simulink model "ulise_internal_v0"  (R2025b)
settings: Solver=FixedStepAuto  StartTime=0.0  StopTime=SimSetup.K - 1  FixedStep=1  RelTol=1e-3
InitFcn:
  | InitFcn_ULISE
model workspace (MAT data in the model file):
  Something = 3
undefined symbols (not defined in the file): SimSetup, System, V
libraries: SignalEditorBlockLib x1
settings Model: Creator=savan  LastModifiedBy=daniellawson
settings DebuggingCC: AlgebraicLoopMsg=none

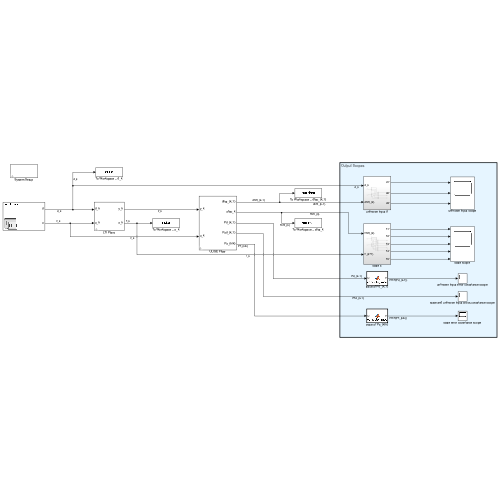
[thumbnail: Simulink's stored preview of the top-level diagram]
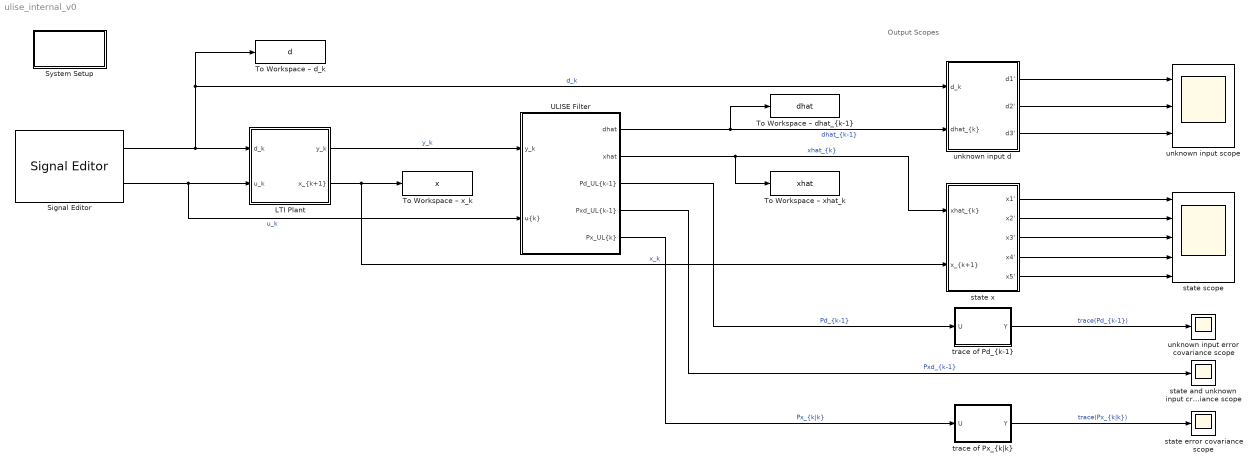
== system ulise_internal_v0 ==
  note: Output Scopes
  LTI Plant : Subsystem  mask{A=System.A, B=System.B, C=System.C, D=System.D, G=System.G, H=System.H, Q=System.Q, R=System.R, InitialState=System.x0, Ts=SimSetup.Ts}
      mask prompts: InitialState "Initial state x_0:"; Ts "Sample Time (-1 for Inherited):"
      mask help:
      | Simulate the states and measurements of a discrete-time, time-invariant linear system of the form:
      |
      | x_{k+1} = A x_k + B u_k + G d_k + w_k,
      | y_k = C x_k + D u_k + H d_k + v_k
      |
      | where x_k is the state vector, u_k is known input vector, d_k is the unknown input vector, y_k is the measurement output vector, w_k is the process noise vector, v_k is the measurement noise vector.
      |
      | Both process noise w_k and measurement noise v_k are zero-mean and uncorrelated, with covariances Q (n-by-n) and R (l-by-l), repsectively.
      mask Help: file:///Users/daniellawson/Documents/Co-op3/Projects/SISE/html/LTI_Plant_Block_overview.html
      mask TypeOptions A: A*x_k multipliation/Gain
      mask TypeOptions B: B*u_k multipliation/Gain
      mask TypeOptions C: C*x_k multipliation/Gain
      mask TypeOptions D: D*u_k multipliation/Gain
      mask TypeOptions G: G*d_k multipliation/Gain
      mask TypeOptions H: H*d_k multipliation/Gain
      mask TypeOptions InitialState: x_{k-1} Delay/InitialCondition
      mask DialogControl DescGroupVar Prompt: Plant
      mask DialogControl ModelParameterContainer Prompt: Model Parameters
      mask DialogControl LTISystemModelContainer Prompt: System Matrices
      mask DialogControl LTISystemNoiseParameters Prompt: Noise Matrices
      mask DialogControl InitialConditions Prompt: Initial Conditions
      mask DialogControl SimulationParameters Prompt: Simulation Paramaters
      mask Display:
      | % Inputs
      | port_label('input', 2, 'u_k');
      | port_label('input', 1, 'd_k');
      | 
      | % Outputs
      | port_label('output', 2, 'x_k');
      | port_label('output', 1, 'y_k');
  Signal Editor : SignalEditorBlockLib/Signal Editor  FileName=ULISE_default_signals.mat  ActiveScenario=input_data  ActiveSignal=d  IsBus=off  OutputBusObjectStr=Bus: BusObject  SampleTime=SimSetup.Ts  Interpolate=off  ZeroCross=off  OutputAfterFinalValue=Holding final value  Unit=inherit  PreserveSignalName=on  ApplySigPropsToAllScenarios=off  ApplySigPropsToAllSignals=off  SignalPropertySource=Signal data in MAT file
  System Setup : Subsystem
      mask help: Describes the files needed to be initialized to use the *LTI Plant* and *ULISE Filter* blocks.
      mask DialogControl ActionsGroupVar Prompt: Actions
      mask DialogControl InitFcnULISEControl Prompt: Open InitFcn_ULISE
      mask DialogControl InitFcnULISEControl Callback: open("./Examples/Simulink/ulise_callbacks/InitFcn_ULISE.m");
  To Workspace – d_k : ToWorkspace  VariableName=d  SaveFormat=Timeseries  SampleTime=-1
  "To Workspace – dhat_{k-1}" : ToWorkspace  VariableName=dhat  SaveFormat=Timeseries  SampleTime=-1
  To Workspace – x_k : ToWorkspace  VariableName=x  SaveFormat=Timeseries  SampleTime=-1
  To Workspace – xhat_k : ToWorkspace  VariableName=xhat  SaveFormat=Timeseries  SampleTime=-1
  ULISE Filter : Subsystem  mask{A=System.A, B=System.B, C=System.C, D=System.D, G=System.G, H=System.H, Q=System.Q, R=System.R, InitialConditionStateEstimate=System.xhat0, InitialConditionStateCov=System.P_x0, Ts=SimSetup.Ts}
      mask prompts: InitialConditionStateEstimate "Initial State Estimate xhat_0:"; InitialConditionStateCov "Initial State Error Covariance Px_0:"; Ts "Sample time (-1 for Inherited):"
      mask help:
      | Estimates the states and unknown inputs of a discrete-time, time-invariant linear system. The states are estimated with a zero-step delay, while the unknown inputs are estimated with a one-step delay.
      |
      | Note: All parameters *must* match the parameters from the LTI Plant Block.
      mask init:
      | %% SVD of H
      | r = rank(H);
      | [U,S,V] = svd(H);
      | U1      = U(:, 1:r); 
      | U2      = U(:, r+1:end);
      | Sigma   = S(1:r, 1:r);
      | V1      = V(:, 1:r);
      | V2      = V(:, r+1:end);
      | 
      | %% Check Assumptions (i) and (ii)
      | 
      | n = size(A,1);
      | p = size(G,2);
      | 
      | if license("test", "Control_Toolbox")
      |     t_zeros = tzero(A,G,C,H)
      |     if rank([A,G;C,H]) ~= n+p
      |         error('Error. System is not strongly detectable.')
      |     end
      |     for i = 1:length(t_zeros)
      |         if abs(t_zeros(i))>1
      |             error('Error. System is not strongly detectable.')
      |         end
      |     end
      | else
      |     warning("Control System Toolbox not available. Condition (i) is not checked.")
      | end
      | 
      | T2 = U2';
      | if rank((T2*C)*(G*V2))<p-r
      |     error('Error. Delay greater or equal to 1. See: Yong, S.Z., Zhu, M., and Frazzoli, E. (2015). Simultaneous input and state estimation with a delay. IEEE Conference on Decision and Control, Osaka, Japan, pp. 468-475')
      | end
      mask TypeOptions InitialConditionStateEstimate: xhat_UL{k} Delay/InitialCondition
      mask TypeOptions InitialConditionStateCov: Px_UL{k} Delay/InitialCondition
      mask DialogControl DescGroupVar Prompt: ULISE Filter
      mask DialogControl ParametersContainer Prompt: Model Parameters
      mask DialogControl ULISESystemModelContainers Prompt: System Matrices
      mask DialogControl ULISENoiseParameters Prompt: Noise Matrices
      mask DialogControl Container6 Prompt: Initial Conditions
      mask DialogControl SimulationParameters Prompt: Simulation Parameters
      mask Display:
      | port_label('input', 2, 'u_k');
      | port_label('input', 1, 'y_k');
      | 
      | port_label('output', 1, 'dhat_{k-1}');
      | port_label('output', 2, 'xhat_k');
      | port_label('output', 3, 'Pd_{k-1}');
      | port_label('output', 4, 'Pxd_{k-1}');
      | port_label('output', 5, 'Px_{k|k}');
  state and unknown input cross-covariance scope : Scope
      settings: ActiveDisplayYMinimum=-5.5275007578366324E+6  ActiveDisplayYMaximum=947500.93266973447
  state error covariance scope : Scope
      settings: ActiveDisplayYMinimum=-621249.98507447576  ActiveDisplayYMaximum=5.5912518070209688E+6  DataLoggingVariableName=ScopeData2
  state scope : Scope  NumInputPorts=5
      settings: ActiveDisplayString=5  ActiveDisplayYMinimum=-0.046170913451183529  ActiveDisplayYMaximum=0.12860695128957148  YLabel=x_5  DataLoggingVariableName=ScopeData7
  state x : Subsystem
  "trace of Pd_{k-1}" : MATLAB Function  TreatAsAtomicUnit=on
  "trace of Px_{k|k}" : MATLAB Function  TreatAsAtomicUnit=on
  unknown input d : Subsystem
  unknown input error covariance scope : Scope
      settings: ActiveDisplayYMinimum=-632500.05670639849  ActiveDisplayYMaximum=5.6925026344334474E+6
  unknown input scope : Scope  NumInputPorts=3
      settings: ActiveDisplayString=3  ActiveDisplayYMinimum=-4.87615367917137  ActiveDisplayYMaximum=4.9009644571376381  YLabel=d_3  DataLoggingVariableName=ScopeData8
  wires:
  ULISE Filter/1(dhat) -> "To Workspace – dhat_{k-1}"/1, unknown input d/2("dhat_{k}")  "dhat_{k-1}"
  Signal Editor/2 -> ULISE Filter/2("u{k}"), LTI Plant/2(u_k)  "u_k"
  Signal Editor/1 -> To Workspace – d_k/1, unknown input d/1(d_k), LTI Plant/1(d_k)  "d_k"
  unknown input d/3(d3') -> unknown input scope/3
  state x/1(x1') -> state scope/1
  state x/3(x3') -> state scope/3
  state x/2(x2') -> state scope/2
  LTI Plant/1(y_k) -> ULISE Filter/1(y_k)  "y_k"
  state x/5(x5') -> state scope/5
  LTI Plant/2("x_{k+1}") -> To Workspace – x_k/1, state x/2("x_{k+1}")  "x_k"
  ULISE Filter/2(xhat) -> To Workspace – xhat_k/1, state x/1("xhat_{k}")  "xhat_{k}"
  unknown input d/1(d1') -> unknown input scope/1
  unknown input d/2(d2') -> unknown input scope/2
  state x/4(x4') -> state scope/4
  ULISE Filter/3("Pd_UL{k-1}") -> "trace of Pd_{k-1}"/1(U)  "Pd_{k-1}"
  ULISE Filter/4("Pxd_UL{k-1}") -> state and unknown input cross-covariance scope/1  "Pxd_{k-1}"
  ULISE Filter/5("Px_UL{k}") -> "trace of Px_{k|k}"/1(U)  "Px_{k|k}"
  "trace of Px_{k|k}"/1(Y) -> state error covariance scope/1  "trace(Px_{k|k})"
  "trace of Pd_{k-1}"/1(Y) -> unknown input error covariance scope/1  "trace(Pd_{k-1})"

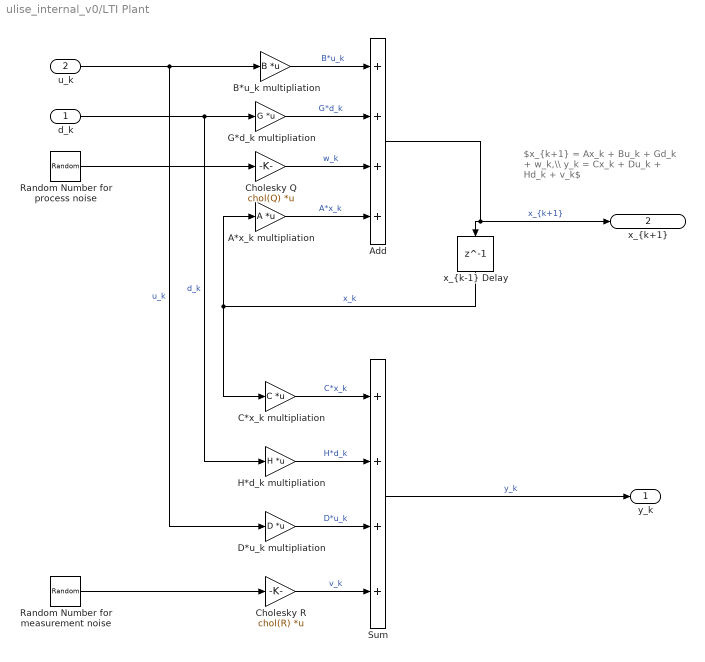
== system ulise_internal_v0/LTI Plant ==
  note: $x_{k+1} = Ax_k + Bu_k + Gd_k + w_k,\\ y_k = Cx_k + Du_k + Hd_k + v_k$
  d_k : Inport
  u_k : Inport  Port=2
  A*x_k multipliation : Gain  Gain=A  Multiplication=Matrix(K*u)
  Add : Sum  Inputs=++++
  B*u_k multipliation : Gain  Gain=B  Multiplication=Matrix(K*u)
  C*x_k multipliation : Gain  Gain=C  Multiplication=Matrix(K*u)
  "Cholesky Q " : Gain  Gain=chol(Q)  Multiplication=Matrix(K*u)
  Cholesky R : Gain  Gain=chol(R)  Multiplication=Matrix(K*u)
  D*u_k multipliation : Gain  Gain=D  Multiplication=Matrix(K*u)
  G*d_k multipliation : Gain  Gain=G  Multiplication=Matrix(K*u)
  H*d_k multipliation : Gain  Gain=H  Multiplication=Matrix(K*u)
  Random Number for measurement noise : RandomNumber  Mean=zeros(size(R,1),1)  Variance=ones(size(R,1),1)  SampleTime=SimSetup.Ts  VectorParams1D=off
  Random Number for process noise : RandomNumber  Mean=zeros(size(Q,1),1)  Variance=ones(size(Q,1),1)  SampleTime=SimSetup.Ts  VectorParams1D=off
  Sum : Sum  Inputs=++++
  "x_{k-1} Delay" : Delay  DelayLength=1  InitialCondition=InitialState
  y_k : Outport
  "x_{k+1}" : Outport  Port=2
  wires:
  D*u_k multipliation/1 -> Sum/3  "D*u_k"
  H*d_k multipliation/1 -> Sum/2  "H*d_k"
  G*d_k multipliation/1 -> Add/2  "G*d_k"
  C*x_k multipliation/1 -> Sum/1  "C*x_k"
  Sum/1 -> y_k/1  "y_k"
  "x_{k-1} Delay"/1 -> A*x_k multipliation/1, C*x_k multipliation/1  "x_k"
  B*u_k multipliation/1 -> Add/1  "B*u_k"
  Add/1 -> "x_{k+1}"/1, "x_{k-1} Delay"/1  "x_{k+1}"
  A*x_k multipliation/1 -> Add/4  "A*x_k"
  d_k/1 -> H*d_k multipliation/1, G*d_k multipliation/1  "d_k"
  u_k/1 -> D*u_k multipliation/1, B*u_k multipliation/1  "u_k"
  Random Number for process noise/1 -> "Cholesky Q "/1
  "Cholesky Q "/1 -> Add/3  "w_k"
  Random Number for measurement noise/1 -> Cholesky R/1
  Cholesky R/1 -> Sum/4  "v_k"

== system ulise_internal_v0/System Setup ==
  note: Edit Initialization Script

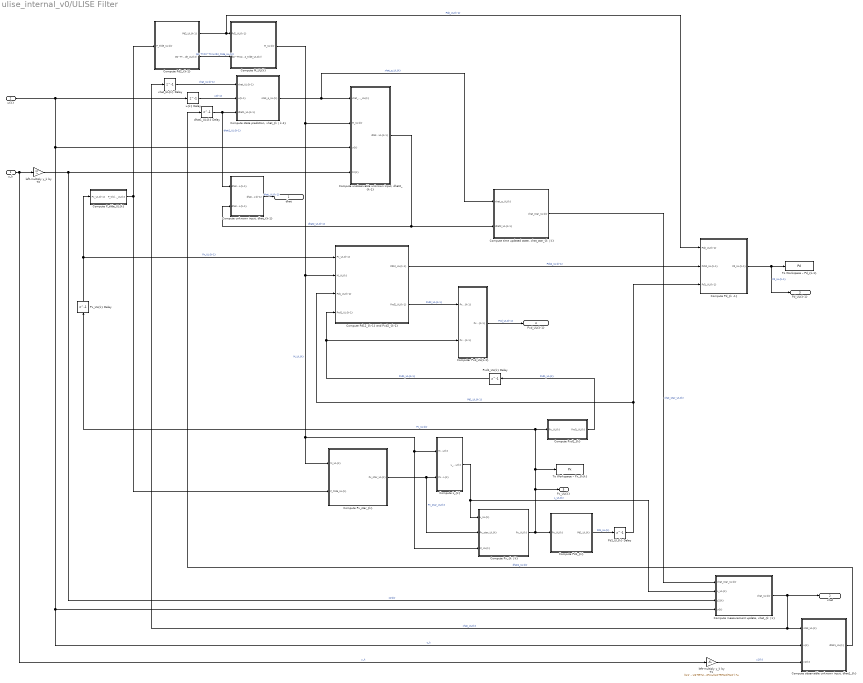
== system ulise_internal_v0/ULISE Filter ==
  y_k : Inport
  "u{k}" : Inport  Port=2
  "Compute L_{k}" : Subsystem
  "Compute M_UL{k}" : Subsystem
  "Compute P_tilde_UL{k}" : Subsystem
  "Compute Pd12_{k-1} and Pxd2_{k-1}" : Subsystem
  "Compute Pd1_{k}" : Subsystem
  "Compute Pd2_{k-1}" : Subsystem
  "Compute Pd_{k -1}" : Subsystem
  "Compute Px_star_{k}" : Subsystem
  "Compute Px_{k | k}" : Subsystem
  "Compute Pxd1_{k}" : Subsystem
  "Compute measurement update, xhat_{k | k}" : Subsystem
  "Compute observable unknown input, dhat1_{k}" : Subsystem
  "Compute state prediction, xhat_{k | k-1} " : Subsystem
  "Compute time updated state, xhat_star_{k | k}" : Subsystem
  "Compute unknown input, dhat_{k-1}" : Subsystem
  "Compute unobservable unknown input, dhat2_{k-1}" : Subsystem
  "Computer Pxd_UL{k-1}" : Subsystem
  "Pd1_UL{k} Delay" : Delay  DelayLength=1
  "Px_UL{k} Delay" : Delay  DelayLength=1  InitialCondition=InitialConditionStateCov  SampleTime=SimSetup.Ts
  "Pxd1_UL{k} Delay" : Delay  DelayLength=1
  "To Workspace – Pd_{k-1}" : ToWorkspace  VariableName=Pd  SaveFormat=Timeseries  SampleTime=-1
  "To Workspace – Px_{k|k}" : ToWorkspace  VariableName=Px  SaveFormat=Timeseries  SampleTime=-1
  "dhat1_UL{k} Delay" : Delay  DelayLength=1  SampleTime=SimSetup.Ts
  left-multiply y_k by T1 : Gain  Gain=(U1' - U1'*R*U2*inv(U2'*R*U2)*U2')  Multiplication=Matrix(K*u)
  "left-multiply y_k by T2 " : Gain  Gain=U2'  Multiplication=Matrix(K*u)
  "u{k} Delay" : Delay  DelayLength=1  SampleTime=SimSetup.Ts
  "xhat_UL{k} Delay" : Delay  DelayLength=1  InitialCondition=InitialConditionStateEstimate  SampleTime=SimSetup.Ts
  dhat : Outport
  xhat : Outport  Port=2
  "Pd_UL{k-1}" : Outport  Port=3
  "Pxd_UL{k-1}" : Outport  Port=4
  "Px_UL{k}" : Outport  Port=5
  wires:
  "Compute Pxd1_{k}"/1("Pxd1_UL{k}") -> "Pxd1_UL{k} Delay"/1  "Pxd1_UL{k}"
  "Compute state prediction, xhat_{k | k-1} "/1("xhat_p_UL{k}") -> "Compute unobservable unknown input, dhat2_{k-1}"/1("xhat_p_UL{k}"), "Compute time updated state, xhat_star_{k | k}"/1("xhat_p_UL{k}")  "xhat_p_UL{k}"
  y_k/1 -> left-multiply y_k by T1/1, "left-multiply y_k by T2 "/1  "y_k"
  left-multiply y_k by T1/1 -> "Compute observable unknown input, dhat1_{k}"/3("z1{k}")  "z1{k}"
  "Compute Pd12_{k-1} and Pxd2_{k-1}"/1("Pd12_UL{k-1}") -> "Compute Pd_{k -1}"/2("Pd12_UL{k-1}")  "Pd12_UL{k-1}"
  "left-multiply y_k by T2 "/1 -> "Compute unobservable unknown input, dhat2_{k-1}"/4("z2{k}"), "Compute measurement update, xhat_{k | k}"/3("z2{k}")  "z2{k}"
  "Compute Pd12_{k-1} and Pxd2_{k-1}"/2("Pxd2_UL{k-1}") -> "Computer Pxd_UL{k-1}"/1("Pxd2_UL{k-1}")  "Pxd2_UL{k-1}"
  "Pd1_UL{k} Delay"/1 -> "Compute Pd_{k -1}"/3("Pd1_UL{k-1}"), "Compute Pd12_{k-1} and Pxd2_{k-1}"/3("Pd1_UL{k-1}")  "Pd1_UL{k-1}"
  "Compute P_tilde_UL{k}"/1("P_tilde_UL{k}") -> "Compute Px_star_{k}"/2("P_tilde_UL{k}"), "Compute Pd2_{k-1}"/1("P_tilde_UL{k}")
  "Pxd1_UL{k} Delay"/1 -> "Compute Pd12_{k-1} and Pxd2_{k-1}"/4("Pxd1_UL{k-1}"), "Computer Pxd_UL{k-1}"/2("Pxd1_UL{k-1}")  "Pxd1_UL{k-1}"
  "Compute M_UL{k}"/1("M_UL{k}") -> "Compute Px_star_{k}"/1("M_UL{k}"), "Compute L_{k}"/1("M_UL{k}"), "Compute Px_{k | k}"/3("M_UL{k}"), "Compute Pd12_{k-1} and Pxd2_{k-1}"/2("M_UL{k}"), "Compute unobservable unknown input, dhat2_{k-1}"/2("M_UL{k}")  "M_UL{k}"
  "Compute Px_star_{k}"/1("Px_star_UL{k}") -> "Compute Px_{k | k}"/2("Px_star_UL{k}"), "Compute L_{k}"/2("Px_star_UL{k}")  "Px_star_UL{k}"
  "Compute Px_{k | k}"/1("Px_UL{k}") -> "Compute Pd1_{k}"/1("Px_UL{k}"), "Px_UL{k}"/1, "Compute Pxd1_{k}"/1("Px_UL{k}"), "Px_UL{k} Delay"/1, "To Workspace – Px_{k|k}"/1  "Px_UL{k}"
  "Compute unknown input, dhat_{k-1}"/1("dhat_UL{k-1}") -> dhat/1  "dhat_UL{k-1}"
  "Compute measurement update, xhat_{k | k}"/1("xhat_UL{k}") -> xhat/1, "xhat_UL{k} Delay"/1, "Compute observable unknown input, dhat1_{k}"/1("xhat_UL{k}")  "xhat_UL{k}"
  "Computer Pxd_UL{k-1}"/1("Pxd_UL{k-1}") -> "Pxd_UL{k-1}"/1  "Pxd_UL{k-1}"
  "Compute Pd2_{k-1}"/1("Pd2_UL{k-1}") -> "Compute Pd_{k -1}"/1("Pd2_UL{k-1}"), "Compute M_UL{k}"/1("Pd2_UL{k-1}")  "Pd2_UL{k-1}"
  "Compute unobservable unknown input, dhat2_{k-1}"/1("dhat2_UL{k-1}") -> "Compute unknown input, dhat_{k-1}"/2("dhat2_UL{k-1}"), "Compute time updated state, xhat_star_{k | k}"/2("dhat2_UL{k-1}")  "dhat2_UL{k-1}"
  "Compute observable unknown input, dhat1_{k}"/1("dhat1_UL{k}") -> "dhat1_UL{k} Delay"/1  "dhat1_UL{k}"
  "dhat1_UL{k} Delay"/1 -> "Compute state prediction, xhat_{k | k-1} "/3("dhat1_UL{k-1}"), "Compute unknown input, dhat_{k-1}"/1("dhat1_UL{k-1}")  "dhat1_UL{k-1}"
  "xhat_UL{k} Delay"/1 -> "Compute state prediction, xhat_{k | k-1} "/1("xhat_UL{k-1}")  "xhat_UL{k-1}"
  "Px_UL{k} Delay"/1 -> "Compute P_tilde_UL{k}"/1("Px_UL{k-1}"), "Compute Pd12_{k-1} and Pxd2_{k-1}"/1("Px_UL{k-1}")  "Px_UL{k-1}"
  "Compute Pd1_{k}"/1("Pd1_UL{k}") -> "Pd1_UL{k} Delay"/1  "Pd1_UL{k}"
  "Compute Pd2_{k-1}"/2("G2^T*C2^T*inv(R2_tilde_UL{k})") -> "Compute M_UL{k}"/2("G2^T*C2^T*inv(R2_tilde_UL{k})")  "G2^T*C2^T*inv(R2_tilde_UL{k})"
  "Compute time updated state, xhat_star_{k | k}"/1("xhat_star_UL{k}") -> "Compute measurement update, xhat_{k | k}"/1("xhat_star_UL{k}")  "xhat_star_UL{k}"
  "u{k}"/1 -> "Compute observable unknown input, dhat1_{k}"/2("u{k}"), "Compute measurement update, xhat_{k | k}"/4("u{k}"), "Compute unobservable unknown input, dhat2_{k-1}"/3("u{k}"), "u{k} Delay"/1  "u_k"
  "Compute L_{k}"/1("L_UL{k}") -> "Compute Px_{k | k}"/1("L_UL{k}"), "Compute measurement update, xhat_{k | k}"/2("L_UL{k}")  "L_UL{k}"
  "Compute Pd_{k -1}"/1("Pd_UL{k-1}") -> "Pd_UL{k-1}"/1, "To Workspace – Pd_{k-1}"/1  "Pd_UL{k-1}"
  "u{k} Delay"/1 -> "Compute state prediction, xhat_{k | k-1} "/2("u{k-1}")  "u{k-1}"

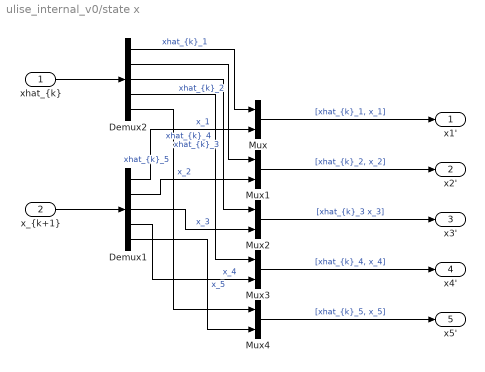
== system ulise_internal_v0/state x ==
  "xhat_{k}" : Inport
  "x_{k+1}" : Inport  Port=2
  Demux1 : Demux  Outputs=5
  Demux2 : Demux  Outputs=5
  Mux{,1..4} (5 alike) : Mux  Inputs=2
  x1' : Outport
  x2' : Outport  Port=2
  x3' : Outport  Port=3
  x4' : Outport  Port=4
  x5' : Outport  Port=5
  wires:
  Mux/1 -> x1'/1  "[xhat_{k}_1, x_1]"
  "xhat_{k}"/1 -> Demux2/1
  Mux4/1 -> x5'/1  "[xhat_{k}_5, x_5]"
  Mux2/1 -> x3'/1  "[xhat_{k}_3 x_3]"
  Demux1/4 -> Mux3/2  "x_4"
  Mux3/1 -> x4'/1  "[xhat_{k}_4, x_4]"
  Mux1/1 -> x2'/1  "[xhat_{k}_2, x_2]"
  Demux1/2 -> Mux1/2  "x_2"
  Demux1/3 -> Mux2/2  "x_3"
  Demux2/5 -> Mux4/1  "xhat_{k}_5"
  Demux2/1 -> Mux/1  "xhat_{k}_1"
  Demux2/4 -> Mux3/1  "xhat_{k}_4"
  Demux2/2 -> Mux1/1  "xhat_{k}_2"
  "x_{k+1}"/1 -> Demux1/1
  Demux1/5 -> Mux4/2  "x_5"
  Demux2/3 -> Mux2/1  "xhat_{k}_3"
  Demux1/1 -> Mux/2  "x_1"

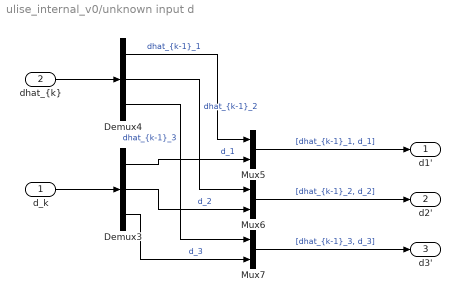
== system ulise_internal_v0/unknown input d ==
  d_k : Inport
  "dhat_{k}" : Inport  Port=2
  Demux3 : Demux  Outputs=3
  Demux4 : Demux  Outputs=3
  Mux5 : Mux  Inputs=2
  Mux6 : Mux  Inputs=2
  Mux7 : Mux  Inputs=2
  d1' : Outport
  d2' : Outport  Port=2
  d3' : Outport  Port=3
  wires:
  Mux6/1 -> d2'/1  "[dhat_{k-1}_2, d_2]"
  d_k/1 -> Demux3/1
  Mux7/1 -> d3'/1  "[dhat_{k-1}_3, d_3]"
  Demux3/3 -> Mux7/2  "d_3"
  Demux4/1 -> Mux5/1  "dhat_{k-1}_1"
  Demux4/2 -> Mux6/1  "dhat_{k-1}_2"
  "dhat_{k}"/1 -> Demux4/1
  Mux5/1 -> d1'/1  "[dhat_{k-1}_1, d_1]"
  Demux3/2 -> Mux6/2  "d_2"
  Demux3/1 -> Mux5/2  "d_1"
  Demux4/3 -> Mux7/1  "dhat_{k-1}_3"

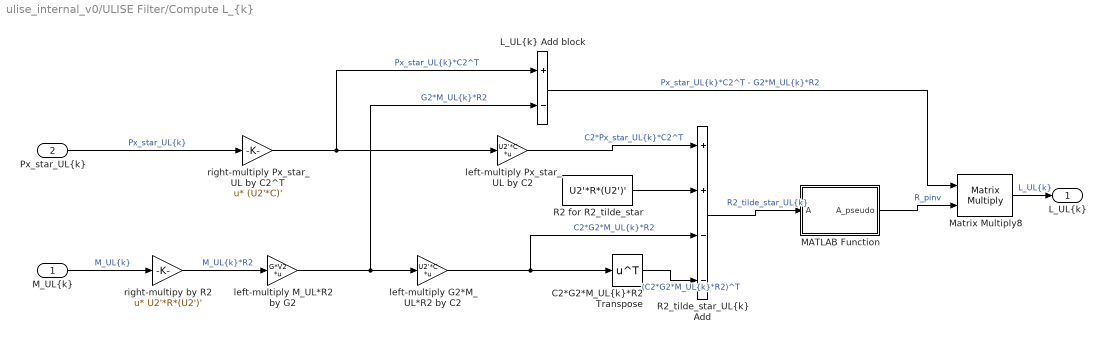
== system ulise_internal_v0/ULISE Filter/Compute L_{k} ==
  "M_UL{k}" : Inport
  "Px_star_UL{k}" : Inport  Port=2
  " R2 for R2_tilde_star" : Constant  Value=U2'*R*(U2')'  VectorParams1D=off  SampleTime=SimSetup.Ts
  "C2*G2*M_UL{k}*R2 Transpose" : Math  Operator=transpose
  "L_UL{k} Add block" : Sum  Inputs=+-
  MATLAB Function : MATLAB Function  TreatAsAtomicUnit=on
  Matrix Multiply8 : Product  Multiplication=Matrix(*)
  "R2_tilde_star_UL{k} Add" : Sum  Inputs=++--
  left-multiply Px_star_UL by C2 : Gain  Gain=U2'*C  Multiplication=Matrix(K*u)
  left-multiply G2*M_UL*R2 by C2 : Gain  Gain=U2'*C  Multiplication=Matrix(K*u)
  left-multiply M_UL*R2 by G2 : Gain  Gain=G*V2  Multiplication=Matrix(K*u)
  "right-multiply Px_star_UL by C2^T " : Gain  Gain=(U2'*C)'  Multiplication=Matrix(u*K)
  right-multipy by R2 : Gain  Gain=U2'*R*(U2')'  Multiplication=Matrix(u*K)
  "L_UL{k}" : Outport
  wires:
  right-multipy by R2/1 -> left-multiply M_UL*R2 by G2/1  "M_UL{k}*R2"
  "Px_star_UL{k}"/1 -> "right-multiply Px_star_UL by C2^T "/1  "Px_star_UL{k}"
  Matrix Multiply8/1 -> "L_UL{k}"/1  "L_UL{k}"
  "right-multiply Px_star_UL by C2^T "/1 -> "L_UL{k} Add block"/1, left-multiply Px_star_UL by C2/1  "Px_star_UL{k}*C2^T"
  left-multiply M_UL*R2 by G2/1 -> left-multiply G2*M_UL*R2 by C2/1, "L_UL{k} Add block"/2  "G2*M_UL{k}*R2"
  "R2_tilde_star_UL{k} Add"/1 -> MATLAB Function/1(A)  "R2_tilde_star_UL{k}"
  left-multiply G2*M_UL*R2 by C2/1 -> "R2_tilde_star_UL{k} Add"/3, "C2*G2*M_UL{k}*R2 Transpose"/1  "C2*G2*M_UL{k}*R2"
  "L_UL{k} Add block"/1 -> Matrix Multiply8/1  "Px_star_UL{k}*C2^T - G2*M_UL{k}*R2"
  " R2 for R2_tilde_star"/1 -> "R2_tilde_star_UL{k} Add"/2
  "M_UL{k}"/1 -> right-multipy by R2/1  "M_UL{k}"
  left-multiply Px_star_UL by C2/1 -> "R2_tilde_star_UL{k} Add"/1  "C2*Px_star_UL{k}*C2^T"
  "C2*G2*M_UL{k}*R2 Transpose"/1 -> "R2_tilde_star_UL{k} Add"/4  "(C2*G2*M_UL{k}*R2)^T"
  MATLAB Function/1(A_pseudo) -> Matrix Multiply8/2  "R_pinv"

== system ulise_internal_v0/ULISE Filter/Compute M_UL{k} ==
  "Pd2_UL{k-1}" : Inport
  "G2^T*C2^T*inv(R2_tilde_UL{k})" : Inport  Port=2
  Matrix Multiply : Product  Multiplication=Matrix(*)
  "M_UL{k}" : Outport
  wires:
  "G2^T*C2^T*inv(R2_tilde_UL{k})"/1 -> Matrix Multiply/2  "G2^T*C2^T*inv(R2_tilde_UL{k})"
  Matrix Multiply/1 -> "M_UL{k}"/1  "M_UL{k}"
  "Pd2_UL{k-1}"/1 -> Matrix Multiply/1  "Pd2_UL{k-1}"

== system ulise_internal_v0/ULISE Filter/Compute P_tilde_UL{k} ==
  "Px_UL{k-1}" : Inport
  Add Qhat : Sum
  Qhat : Constant  Value=G*V1*pinv(Sigma)*((U1' - U1'*R*U2*inv(U2'*R*U2)*U2')*R*(U1' - U1'*R*U2*inv(U2'*R*U2)*U2')')*pinv(Sigma)'*(G*V1)' + Q  VectorParams1D=off  SampleTime=SimSetup.Ts
  left-multiply by Ahat : Gain  Gain=A - G*V1*pinv(Sigma)*((U1' - U1'*R*U2*inv(U2'*R*U2)*U2')*C)  Multiplication=Matrix(K*u)
  right-multiply by Ahat^T : Gain  Gain=(A - G*V1*pinv(Sigma)*((U1' - U1'*R*U2*inv(U2'*R*U2)*U2')*C))'  Multiplication=Matrix(u*K)
  "P_tilde_UL{k}" : Outport
  wires:
  Add Qhat/1 -> "P_tilde_UL{k}"/1  "P_tilde_UL{k}"
  "Px_UL{k-1}"/1 -> right-multiply by Ahat^T/1  "Px_UL{k-1}"
  right-multiply by Ahat^T/1 -> left-multiply by Ahat/1  "Px_UL{k-1}*Ahat^T"
  left-multiply by Ahat/1 -> Add Qhat/1  "Ahat*Px_UL{k-1}*Ahat^T"
  Qhat/1 -> Add Qhat/2  "Qhat"

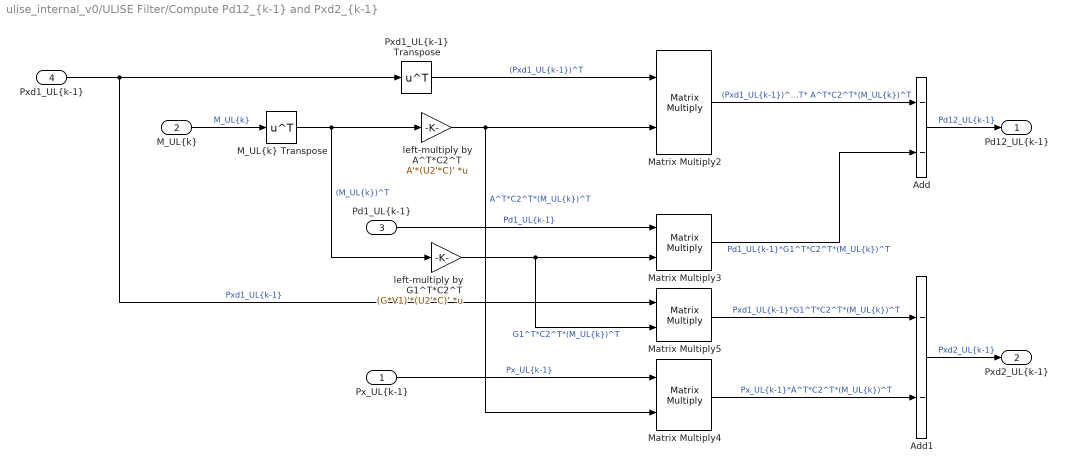
== system ulise_internal_v0/ULISE Filter/Compute Pd12_{k-1} and Pxd2_{k-1} ==
  "Px_UL{k-1}" : Inport
  "M_UL{k}" : Inport  Port=2
  "Pd1_UL{k-1}" : Inport  Port=3
  "Pxd1_UL{k-1}" : Inport  Port=4
  Add : Sum  Inputs=--
  Add1 : Sum  Inputs=--
  "M_UL{k} Transpose" : Math  Operator=transpose
  Matrix Multiply{2..5} (4 alike) : Product  Multiplication=Matrix(*)
  "Pxd1_UL{k-1} Transpose" : Math  Operator=transpose
  left-multiply by A^T*C2^T : Gain  Gain=A'*(U2'*C)'  Multiplication=Matrix(K*u)
  left-multiply by G1^T*C2^T : Gain  Gain=(G*V1)'*(U2'*C)'  Multiplication=Matrix(K*u)
  "Pd12_UL{k-1}" : Outport
  "Pxd2_UL{k-1}" : Outport  Port=2
  wires:
  Add1/1 -> "Pxd2_UL{k-1}"/1  "Pxd2_UL{k-1}"
  left-multiply by A^T*C2^T/1 -> Matrix Multiply2/2, Matrix Multiply4/2  "A^T*C2^T*(M_UL{k})^T"
  Matrix Multiply5/1 -> Add1/1  "Pxd1_UL{k-1}*G1^T*C2^T*(M_UL{k})^T"
  left-multiply by G1^T*C2^T/1 -> Matrix Multiply3/2, Matrix Multiply5/2  "G1^T*C2^T*(M_UL{k})^T"
  Matrix Multiply3/1 -> Add/2  "Pd1_UL{k-1}*G1^T*C2^T*(M_UL{k})^T"
  "M_UL{k}"/1 -> "M_UL{k} Transpose"/1  "M_UL{k}"
  "Pd1_UL{k-1}"/1 -> Matrix Multiply3/1  "Pd1_UL{k-1}"
  Add/1 -> "Pd12_UL{k-1}"/1  "Pd12_UL{k-1}"
  Matrix Multiply4/1 -> Add1/2  "Px_UL{k-1}*A^T*C2^T*(M_UL{k})^T"
  "Px_UL{k-1}"/1 -> Matrix Multiply4/1  "Px_UL{k-1}"
  Matrix Multiply2/1 -> Add/1  "(Pxd1_UL{k-1})^T* A^T*C2^T*(M_UL{k})^T"
  "Pxd1_UL{k-1} Transpose"/1 -> Matrix Multiply2/1  "(Pxd1_UL{k-1})^T"
  "Pxd1_UL{k-1}"/1 -> "Pxd1_UL{k-1} Transpose"/1, Matrix Multiply5/1  "Pxd1_UL{k-1}"
  "M_UL{k} Transpose"/1 -> left-multiply by G1^T*C2^T/1, left-multiply by A^T*C2^T/1  "(M_UL{k})^T"

== system ulise_internal_v0/ULISE Filter/Compute Pd1_{k} ==
  "Px_UL{k}" : Inport
  "R1 " : Constant  Value=(U1' - U1'*R*U2*inv(U2'*R*U2)*U2')*R*(U1' - U1'*R*U2*inv(U2'*R*U2)*U2')'  VectorParams1D=off  SampleTime=SimSetup.Ts
  "R1_tilde_UL{k} Add" : Sum
  "left-multiply Px_UL{k}*C1^T by C1" : Gain  Gain=(U1' - U1'*R*U2*inv(U2'*R*U2)*U2')*C  Multiplication=Matrix(K*u)
  "left-multiply R1_tilde_UL{k}*M1 by M1" : Gain  Gain=pinv(Sigma)  Multiplication=Matrix(K*u)
  "right-multiply Px_UL{k} by C1^T" : Gain  Gain=((U1' - U1'*R*U2*inv(U2'*R*U2)*U2')*C)'  Multiplication=Matrix(u*K)
  "right-multiply R1_tilde_UL{k} by M1" : Gain  Gain=pinv(Sigma)  Multiplication=Matrix(u*K)
  "Pd1_UL{k}" : Outport
  wires:
  "Px_UL{k}"/1 -> "right-multiply Px_UL{k} by C1^T"/1
  "right-multiply Px_UL{k} by C1^T"/1 -> "left-multiply Px_UL{k}*C1^T by C1"/1  "Px_UL{k}*C1^T"
  "right-multiply R1_tilde_UL{k} by M1"/1 -> "left-multiply R1_tilde_UL{k}*M1 by M1"/1  "R1_tilde_UL{k}*M1"
  "left-multiply R1_tilde_UL{k}*M1 by M1"/1 -> "Pd1_UL{k}"/1  "Pd1_UL{k}"
  "left-multiply Px_UL{k}*C1^T by C1"/1 -> "R1_tilde_UL{k} Add"/1  "C1*Px_UL{k}*C1^T"
  "R1_tilde_UL{k} Add"/1 -> "right-multiply R1_tilde_UL{k} by M1"/1  "R1_tilde_UL{k}"
  "R1 "/1 -> "R1_tilde_UL{k} Add"/2

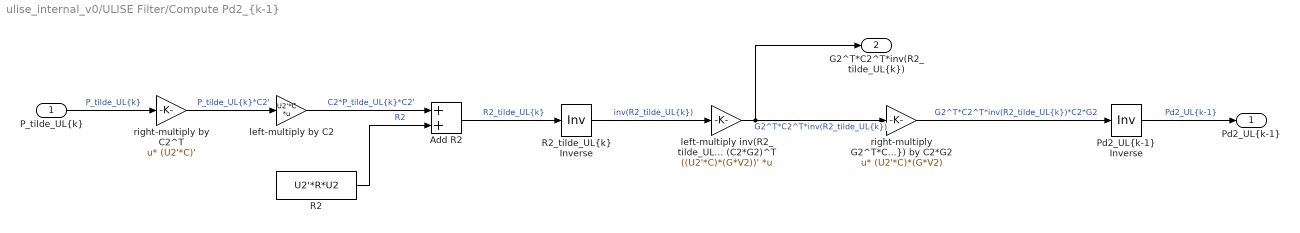
== system ulise_internal_v0/ULISE Filter/Compute Pd2_{k-1} ==
  "P_tilde_UL{k}" : Inport
  Add R2 : Sum
  "Pd2_UL{k-1} Inverse" : Product  Inputs=/  Multiplication=Matrix(*)
  R2 : Constant  Value=U2'*R*U2  VectorParams1D=off  SampleTime=SimSetup.Ts
  "R2_tilde_UL{k} Inverse" : Product  Inputs=/  Multiplication=Matrix(*)
  "left-multiply inv(R2_tilde_UL{k}) by (C2*G2)^T " : Gain  Gain=((U2'*C)*(G*V2))'  Multiplication=Matrix(K*u)
  left-multiply by C2 : Gain  Gain=U2'*C  Multiplication=Matrix(K*u)
  "right-multiply G2^T*C2^T*inv(R2_tilde_UL{k}) by C2*G2" : Gain  Gain=(U2'*C)*(G*V2)  Multiplication=Matrix(u*K)
  right-multiply by C2^T : Gain  Gain=(U2'*C)'  Multiplication=Matrix(u*K)
  "Pd2_UL{k-1}" : Outport
  "G2^T*C2^T*inv(R2_tilde_UL{k})" : Outport  Port=2
  wires:
  left-multiply by C2/1 -> Add R2/1  "C2*P_tilde_UL{k}*C2'"
  "P_tilde_UL{k}"/1 -> right-multiply by C2^T/1  "P_tilde_UL{k}"
  right-multiply by C2^T/1 -> left-multiply by C2/1  "P_tilde_UL{k}*C2'"
  "right-multiply G2^T*C2^T*inv(R2_tilde_UL{k}) by C2*G2"/1 -> "Pd2_UL{k-1} Inverse"/1  "G2^T*C2^T*inv(R2_tilde_UL{k})*C2*G2"
  "R2_tilde_UL{k} Inverse"/1 -> "left-multiply inv(R2_tilde_UL{k}) by (C2*G2)^T "/1  "inv(R2_tilde_UL{k})"
  R2/1 -> Add R2/2  "R2"
  "Pd2_UL{k-1} Inverse"/1 -> "Pd2_UL{k-1}"/1  "Pd2_UL{k-1}"
  Add R2/1 -> "R2_tilde_UL{k} Inverse"/1  "R2_tilde_UL{k}"
  "left-multiply inv(R2_tilde_UL{k}) by (C2*G2)^T "/1 -> "right-multiply G2^T*C2^T*inv(R2_tilde_UL{k}) by C2*G2"/1, "G2^T*C2^T*inv(R2_tilde_UL{k})"/1  "G2^T*C2^T*inv(R2_tilde_UL{k})"

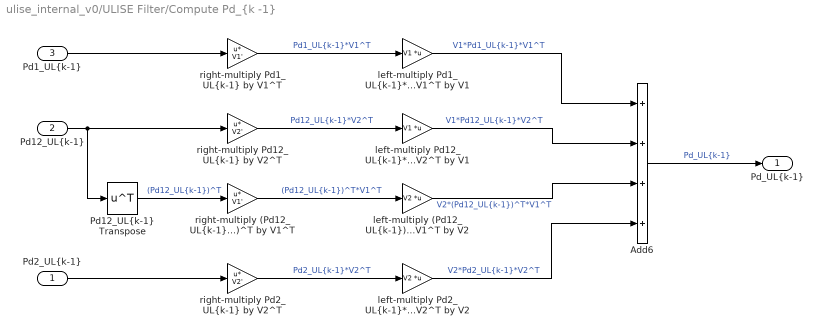
== system ulise_internal_v0/ULISE Filter/Compute Pd_{k -1} ==
  "Pd2_UL{k-1}" : Inport
  "Pd12_UL{k-1}" : Inport  Port=2
  "Pd1_UL{k-1}" : Inport  Port=3
  Add6 : Sum  Inputs=++++
  "Pd12_UL{k-1} Transpose" : Math  Operator=transpose
  "left-multiply (Pd12_UL{k-1})^T*V1^T by V2" : Gain  Gain=V2  Multiplication=Matrix(K*u)
  "left-multiply Pd12_UL{k-1}*V2^T by V1" : Gain  Gain=V1  Multiplication=Matrix(K*u)
  "left-multiply Pd1_UL{k-1}*V1^T by V1" : Gain  Gain=V1  Multiplication=Matrix(K*u)
  "left-multiply Pd2_UL{k-1}*V2^T by V2" : Gain  Gain=V2  Multiplication=Matrix(K*u)
  "right-multiply (Pd12_UL{k-1})^T by V1^T" : Gain  Gain=V1'  Multiplication=Matrix(u*K)
  "right-multiply Pd12_UL{k-1} by V2^T" : Gain  Gain=V2'  Multiplication=Matrix(u*K)
  "right-multiply Pd1_UL{k-1} by V1^T" : Gain  Gain=V1'  Multiplication=Matrix(u*K)
  "right-multiply Pd2_UL{k-1} by V2^T" : Gain  Gain=V2'  Multiplication=Matrix(u*K)
  "Pd_UL{k-1}" : Outport
  wires:
  "Pd2_UL{k-1}"/1 -> "right-multiply Pd2_UL{k-1} by V2^T"/1
  "Pd12_UL{k-1}"/1 -> "right-multiply Pd12_UL{k-1} by V2^T"/1, "Pd12_UL{k-1} Transpose"/1
  "left-multiply Pd12_UL{k-1}*V2^T by V1"/1 -> Add6/2  "V1*Pd12_UL{k-1}*V2^T"
  "Pd1_UL{k-1}"/1 -> "right-multiply Pd1_UL{k-1} by V1^T"/1
  "left-multiply Pd2_UL{k-1}*V2^T by V2"/1 -> Add6/4  "V2*Pd2_UL{k-1}*V2^T"
  "right-multiply Pd12_UL{k-1} by V2^T"/1 -> "left-multiply Pd12_UL{k-1}*V2^T by V1"/1  "Pd12_UL{k-1}*V2^T"
  "left-multiply Pd1_UL{k-1}*V1^T by V1"/1 -> Add6/1  "V1*Pd1_UL{k-1}*V1^T"
  "right-multiply (Pd12_UL{k-1})^T by V1^T"/1 -> "left-multiply (Pd12_UL{k-1})^T*V1^T by V2"/1  "(Pd12_UL{k-1})^T*V1^T"
  Add6/1 -> "Pd_UL{k-1}"/1  "Pd_UL{k-1}"
  "right-multiply Pd1_UL{k-1} by V1^T"/1 -> "left-multiply Pd1_UL{k-1}*V1^T by V1"/1  "Pd1_UL{k-1}*V1^T"
  "right-multiply Pd2_UL{k-1} by V2^T"/1 -> "left-multiply Pd2_UL{k-1}*V2^T by V2"/1  "Pd2_UL{k-1}*V2^T"
  "left-multiply (Pd12_UL{k-1})^T*V1^T by V2"/1 -> Add6/3  "V2*(Pd12_UL{k-1})^T*V1^T"
  "Pd12_UL{k-1} Transpose"/1 -> "right-multiply (Pd12_UL{k-1})^T by V1^T"/1  "(Pd12_UL{k-1})^T"

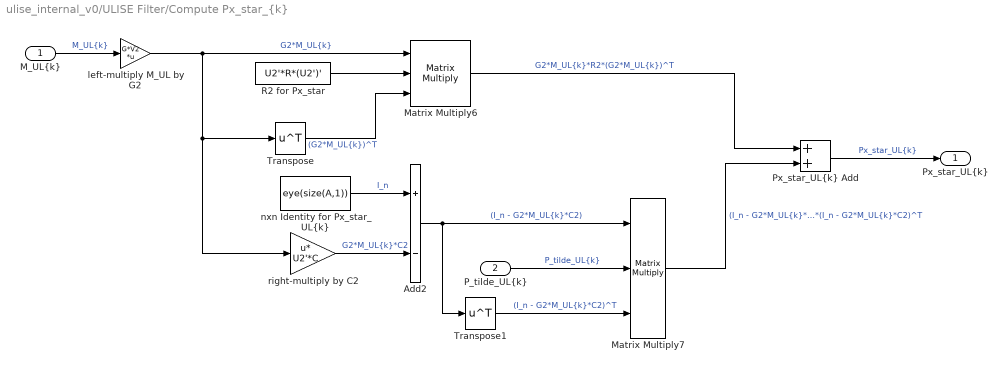
== system ulise_internal_v0/ULISE Filter/Compute Px_star_{k} ==
  "M_UL{k}" : Inport
  "P_tilde_UL{k}" : Inport  Port=2
  " R2 for Px_star" : Constant  Value=U2'*R*(U2')'  SampleTime=SimSetup.Ts
  Add2 : Sum  Inputs=+-
  Matrix Multiply6 : Product  Inputs=3  Multiplication=Matrix(*)
  Matrix Multiply7 : Product  Inputs=3  Multiplication=Matrix(*)
  "Px_star_UL{k} Add" : Sum
  Transpose : Math  Operator=transpose
  Transpose1 : Math  Operator=transpose
  left-multiply M_UL by G2 : Gain  Gain=G*V2  Multiplication=Matrix(K*u)
  "nxn Identity for Px_star_UL{k}" : Constant  Value=eye(size(A,1))  VectorParams1D=off  SampleTime=SimSetup.Ts
  right-multiply by C2 : Gain  Gain=U2'*C  Multiplication=Matrix(u*K)
  "Px_star_UL{k}" : Outport
  wires:
  right-multiply by C2/1 -> Add2/2  "G2*M_UL{k}*C2"
  left-multiply M_UL by G2/1 -> right-multiply by C2/1, Transpose/1, Matrix Multiply6/1  "G2*M_UL{k}"
  Transpose1/1 -> Matrix Multiply7/3  "(I_n - G2*M_UL{k}*C2)^T"
  Matrix Multiply7/1 -> "Px_star_UL{k} Add"/2  "(I_n - G2*M_UL{k}*C2)*P_tilde*(I_n - G2*M_UL{k}*C2)^T"
  " R2 for Px_star"/1 -> Matrix Multiply6/2
  "M_UL{k}"/1 -> left-multiply M_UL by G2/1  "M_UL{k}"
  "P_tilde_UL{k}"/1 -> Matrix Multiply7/2  "P_tilde_UL{k}"
  "Px_star_UL{k} Add"/1 -> "Px_star_UL{k}"/1  "Px_star_UL{k}"
  Add2/1 -> Transpose1/1, Matrix Multiply7/1  "(I_n - G2*M_UL{k}*C2)"
  "nxn Identity for Px_star_UL{k}"/1 -> Add2/1  "I_n"
  Transpose/1 -> Matrix Multiply6/3  "(G2*M_UL{k})^T"
  Matrix Multiply6/1 -> "Px_star_UL{k} Add"/1  "G2*M_UL{k}*R2*(G2*M_UL{k})^T"

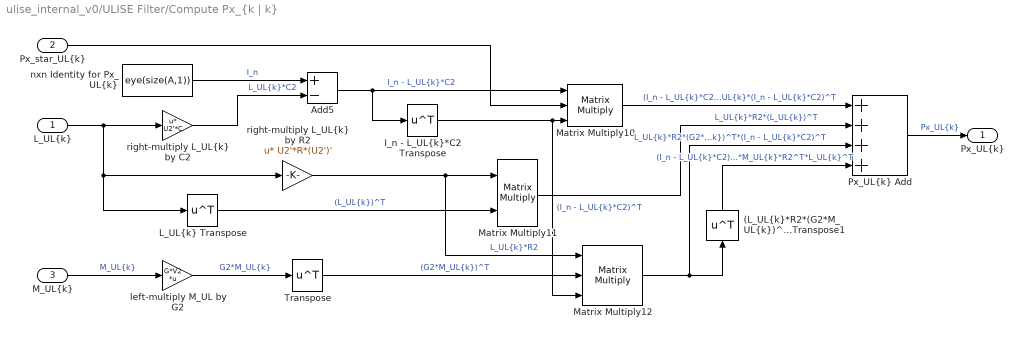
== system ulise_internal_v0/ULISE Filter/Compute Px_{k | k} ==
  "L_UL{k}" : Inport
  "Px_star_UL{k}" : Inport  Port=2
  "M_UL{k}" : Inport  Port=3
  "(L_UL{k}*R2*(G2*M_UL{k})^T*(I_n - L_UL{k}*C2)^T) Transpose1" : Math  Operator=transpose
  Add5 : Sum  Inputs=+-
  "I_n - L_UL{k}*C2 Transpose" : Math  Operator=transpose
  "L_UL{k} Transpose" : Math  Operator=transpose
  Matrix Multiply10 : Product  Inputs=3  Multiplication=Matrix(*)
  Matrix Multiply11 : Product  Multiplication=Matrix(*)
  Matrix Multiply12 : Product  Inputs=3  Multiplication=Matrix(*)
  "Px_UL{k} Add" : Sum  Inputs=++++
  Transpose : Math  Operator=transpose
  left-multiply M_UL by G2 : Gain  Gain=G*V2  Multiplication=Matrix(K*u)
  "nxn Identity for Px_UL{k}" : Constant  Value=eye(size(A,1))  VectorParams1D=off  SampleTime=SimSetup.Ts
  "right-multiply L_UL{k} by C2" : Gain  Gain=U2'*C  Multiplication=Matrix(u*K)
  "right-multiply L_UL{k} by R2" : Gain  Gain=U2'*R*(U2')'  Multiplication=Matrix(u*K)
  "Px_UL{k}" : Outport
  wires:
  "Px_star_UL{k}"/1 -> Matrix Multiply10/2
  "L_UL{k} Transpose"/1 -> Matrix Multiply11/2  "(L_UL{k})^T"
  Add5/1 -> "I_n - L_UL{k}*C2 Transpose"/1, Matrix Multiply10/1  "I_n - L_UL{k}*C2"
  Matrix Multiply10/1 -> "Px_UL{k} Add"/1  "(I_n - L_UL{k}*C2)*Px_star_UL{k}*(I_n - L_UL{k}*C2)^T"
  "Px_UL{k} Add"/1 -> "Px_UL{k}"/1  "Px_UL{k}"
  Matrix Multiply12/1 -> "Px_UL{k} Add"/3, "(L_UL{k}*R2*(G2*M_UL{k})^T*(I_n - L_UL{k}*C2)^T) Transpose1"/1  "L_UL{k}*R2*(G2*M_UL{k})^T*(I_n - L_UL{k}*C2)^T"
  "(L_UL{k}*R2*(G2*M_UL{k})^T*(I_n - L_UL{k}*C2)^T) Transpose1"/1 -> "Px_UL{k} Add"/4  "(I_n - L_UL{k}*C2)*G2*M_UL{k}*R2^T*L_UL{k}^T"
  "right-multiply L_UL{k} by C2"/1 -> Add5/2  "L_UL{k}*C2"
  "L_UL{k}"/1 -> "right-multiply L_UL{k} by C2"/1, "right-multiply L_UL{k} by R2"/1, "L_UL{k} Transpose"/1
  Matrix Multiply11/1 -> "Px_UL{k} Add"/2  "L_UL{k}*R2*(L_UL{k})^T"
  "right-multiply L_UL{k} by R2"/1 -> Matrix Multiply12/1, Matrix Multiply11/1  "L_UL{k}*R2"
  "nxn Identity for Px_UL{k}"/1 -> Add5/1  "I_n"
  "I_n - L_UL{k}*C2 Transpose"/1 -> Matrix Multiply12/3, Matrix Multiply10/3  "(I_n - L_UL{k}*C2)^T"
  "M_UL{k}"/1 -> left-multiply M_UL by G2/1  "M_UL{k}"
  left-multiply M_UL by G2/1 -> Transpose/1  "G2*M_UL{k}"
  Transpose/1 -> Matrix Multiply12/2  "(G2*M_UL{k})^T"

== system ulise_internal_v0/ULISE Filter/Compute Pxd1_{k} ==
  "Px_UL{k}" : Inport
  "right-multiply Px_UL{k} by -C1^T*M1^T" : Gain  Gain=-1*((U1' - U1'*R*U2*inv(U2'*R*U2)*U2')*C)'*(pinv(Sigma))'  Multiplication=Matrix(u*K)
  "Pxd1_UL{k}" : Outport
  wires:
  "Px_UL{k}"/1 -> "right-multiply Px_UL{k} by -C1^T*M1^T"/1
  "right-multiply Px_UL{k} by -C1^T*M1^T"/1 -> "Pxd1_UL{k}"/1  "Pxd1_UL{k}"

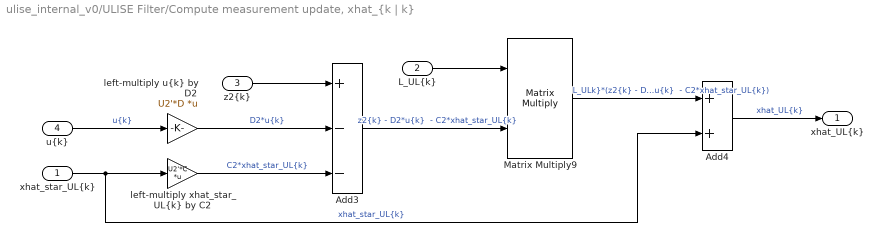
== system ulise_internal_v0/ULISE Filter/Compute measurement update, xhat_{k | k} ==
  "xhat_star_UL{k}" : Inport
  "L_UL{k}" : Inport  Port=2
  "z2{k}" : Inport  Port=3
  "u{k}" : Inport  Port=4
  Add3 : Sum  Inputs=+--
  Add4 : Sum
  Matrix Multiply9 : Product  Multiplication=Matrix(*)
  "left-multiply u{k} by D2" : Gain  Gain=U2'*D  Multiplication=Matrix(K*u)
  "left-multiply xhat_star_UL{k} by C2" : Gain  Gain=U2'*C  Multiplication=Matrix(K*u)
  "xhat_UL{k}" : Outport
  wires:
  "left-multiply xhat_star_UL{k} by C2"/1 -> Add3/3  "C2*xhat_star_UL{k}"
  Add4/1 -> "xhat_UL{k}"/1  "xhat_UL{k}"
  "z2{k}"/1 -> Add3/1
  "xhat_star_UL{k}"/1 -> Add4/2, "left-multiply xhat_star_UL{k} by C2"/1  "xhat_star_UL{k}"
  Matrix Multiply9/1 -> Add4/1  "L_ULk}*(z2{k} - D2*u{k}  - C2*xhat_star_UL{k})"
  "u{k}"/1 -> "left-multiply u{k} by D2"/1  "u{k}"
  "left-multiply u{k} by D2"/1 -> Add3/2  "D2*u{k}"
  "L_UL{k}"/1 -> Matrix Multiply9/1
  Add3/1 -> Matrix Multiply9/2  "z2{k} - D2*u{k}  - C2*xhat_star_UL{k}"

== system ulise_internal_v0/ULISE Filter/Compute observable unknown input, dhat1_{k} ==
  "xhat_UL{k}" : Inport
  "u{k}" : Inport  Port=2
  "z1{k}" : Inport  Port=3
  dhat1 Add block : Sum  Inputs=+--
  left-multiply by M1 : Gain  Gain=pinv(Sigma)  Multiplication=Matrix(K*u)
  "left-multiply u{k} by D1" : Gain  Gain=(U1' - U1'*R*U2*inv(U2'*R*U2)*U2')*D  Multiplication=Matrix(K*u)
  "left-multiply xhat_UL{k} by C1" : Gain  Gain=(U1' - U1'*R*U2*inv(U2'*R*U2)*U2')*C  Multiplication=Matrix(K*u)
  "dhat1_UL{k}" : Outport
  wires:
  "xhat_UL{k}"/1 -> "left-multiply xhat_UL{k} by C1"/1
  left-multiply by M1/1 -> "dhat1_UL{k}"/1  "dhat1_UL{k}"
  "left-multiply u{k} by D1"/1 -> dhat1 Add block/3
  "left-multiply xhat_UL{k} by C1"/1 -> dhat1 Add block/2
  "z1{k}"/1 -> dhat1 Add block/1  "z1{k}"
  "u{k}"/1 -> "left-multiply u{k} by D1"/1
  dhat1 Add block/1 -> left-multiply by M1/1  "z1{k} - C1*xhat_UL{k}  - D1*u{k}"

== system ulise_internal_v0/ULISE Filter/Compute state prediction, xhat_{k | k-1}  ==
  "xhat_UL{k-1}" : Inport
  "u{k-1}" : Inport  Port=2
  "dhat1_UL{k-1}" : Inport  Port=3
  left-multiply by A : Gain  Gain=A  Multiplication=Matrix(K*u)
  left-multiply by B : Gain  Gain=B  Multiplication=Matrix(K*u)
  left-multiply by G1 : Gain  Gain=G*V1  Multiplication=Matrix(K*u)
  "xhat_p_UL{k} Add" : Sum  Inputs=+++
  "xhat_p_UL{k}" : Outport
  wires:
  "dhat1_UL{k-1}"/1 -> left-multiply by G1/1
  left-multiply by B/1 -> "xhat_p_UL{k} Add"/2  "B*u{k-1}"
  left-multiply by A/1 -> "xhat_p_UL{k} Add"/1  "A*xhat_UL{k-1}"
  "u{k-1}"/1 -> left-multiply by B/1
  "xhat_p_UL{k} Add"/1 -> "xhat_p_UL{k}"/1  "xhat_p_UL{k}"
  "xhat_UL{k-1}"/1 -> left-multiply by A/1
  left-multiply by G1/1 -> "xhat_p_UL{k} Add"/3  "G*dhat1_UL{k-1}"

== system ulise_internal_v0/ULISE Filter/Compute time updated state, xhat_star_{k | k} ==
  "xhat_p_UL{k}" : Inport
  "dhat2_UL{k-1}" : Inport  Port=2
  left-multiply by G2 : Gain  Gain=G*V2  Multiplication=Matrix(K*u)
  "xhat_star_UL{k} Add" : Sum
  "xhat_star_UL{k}" : Outport
  wires:
  "dhat2_UL{k-1}"/1 -> left-multiply by G2/1
  "xhat_p_UL{k}"/1 -> "xhat_star_UL{k} Add"/1
  "xhat_star_UL{k} Add"/1 -> "xhat_star_UL{k}"/1  "xhat_star_UL{k}"
  left-multiply by G2/1 -> "xhat_star_UL{k} Add"/2  "G2*dhat2_UL{k-1}"

== system ulise_internal_v0/ULISE Filter/Compute unknown input, dhat_{k-1} ==
  "dhat1_UL{k-1}" : Inport
  "dhat2_UL{k-1}" : Inport  Port=2
  "dhat_UL{k-1} Mux" : Mux  Inputs=2
  left-multiply by V : Gain  Gain=V  Multiplication=Matrix(K*u)
  "dhat_UL{k-1}" : Outport
  wires:
  "dhat2_UL{k-1}"/1 -> "dhat_UL{k-1} Mux"/2
  "dhat1_UL{k-1}"/1 -> "dhat_UL{k-1} Mux"/1
  left-multiply by V/1 -> "dhat_UL{k-1}"/1  "dhat_UL{k-1}"
  "dhat_UL{k-1} Mux"/1 -> left-multiply by V/1  "[dhat1{k-1}; dhat2{k-1}]"

== system ulise_internal_v0/ULISE Filter/Compute unobservable unknown input, dhat2_{k-1} ==
  note: unknown unobservable input estimate at previous time step
  "xhat_p_UL{k}" : Inport
  "M_UL{k}" : Inport  Port=2
  "u{k}" : Inport  Port=3
  "z2{k}" : Inport  Port=4
  Matrix Multiply1 : Product  Multiplication=Matrix(*)
  dhat2 Add : Sum  Inputs=+--
  left-multiply by D2 : Gain  Gain=U2'*D  Multiplication=Matrix(K*u)
  "left-multiply xhat_p_UL{k} by C2" : Gain  Gain=U2'*C  Multiplication=Matrix(K*u)
  "dhat2_UL{k-1}" : Outport
  wires:
  "M_UL{k}"/1 -> Matrix Multiply1/1  "M_UL{k}"
  dhat2 Add/1 -> Matrix Multiply1/2  "z2{k} - C2*xhat_p_UL{k} - D2*u{k}"
  "u{k}"/1 -> left-multiply by D2/1  "u{k}"
  "z2{k}"/1 -> dhat2 Add/1  "z2{k}"
  "left-multiply xhat_p_UL{k} by C2"/1 -> dhat2 Add/2  "C2*xhat_p_UL{k}"
  left-multiply by D2/1 -> dhat2 Add/3  "D2*u{k}"
  Matrix Multiply1/1 -> "dhat2_UL{k-1}"/1  "dhat2_UL{k-1}"
  "xhat_p_UL{k}"/1 -> "left-multiply xhat_p_UL{k} by C2"/1

== system ulise_internal_v0/ULISE Filter/Computer Pxd_UL{k-1} ==
  "Pxd2_UL{k-1}" : Inport
  "Pxd1_UL{k-1}" : Inport  Port=2
  Add : Sum
  "right-multiply Pxd1_UL{k-1} by V1^T" : Gain  Gain=V1'  Multiplication=Matrix(u*K)
  "right-multiply Pxd2_UL{k-1} by V2^T" : Gain  Gain=V2'  Multiplication=Matrix(u*K)
  "Pxd_UL{k-1}" : Outport
  wires:
  "Pxd1_UL{k-1}"/1 -> "right-multiply Pxd1_UL{k-1} by V1^T"/1  "Pxd1_UL{k-1}"
  Add/1 -> "Pxd_UL{k-1}"/1  "Pxd_UL{k-1}"
  "Pxd2_UL{k-1}"/1 -> "right-multiply Pxd2_UL{k-1} by V2^T"/1  "Pxd2_UL{k-1}"
  "right-multiply Pxd2_UL{k-1} by V2^T"/1 -> Add/2
  "right-multiply Pxd1_UL{k-1} by V1^T"/1 -> Add/1

== matlab function ulise_internal_v0/ULISE Filter/Compute L_{k}/MATLAB Function ==
  data: A input; A_pseudo output
function A_pseudo = pseudoinv_fcn(A)
% Computes the Moore–Penrose inverse (A_pseudo) of the input matrix A using
% MATLAB's built-in pinv function.
%
% Input:
%   A - Input matrix of size m x n.
%
% Output:
%   A_pseudo - pseudoinverse of A, of size n x m.

A_pseudo = pinv(A);

== matlab function ulise_internal_v0/trace of Pd_{k-1} ==
  data: U input; Y output
function Y = compute_trace(U)
% COMPUTE_TRACE computes the trace of a square matrix.
%
%   Y = COMPUTE_TRACE(U) computes and returns the trace of the input matrix
%   U. This utility is intended to aid in visualization of covariance
%   matrices.

Y = trace(U);

== matlab function ulise_internal_v0/trace of Px_{k|k} ==
  data: U input; Y output
function Y = compute_trace(U)
% COMPUTE_TRACE computes the trace of a square matrix.
%
%   Y = COMPUTE_TRACE(U) computes and returns the trace of the input matrix
%   U. This utility is intended to aid in visualization of covariance
%   matrices.

Y = trace(U);
